simulink model "PID_validation_3_3_2"  (R2024b)
settings: Solver=FixedStepDiscrete  StartTime=0.0  StopTime=20  FixedStep=0.001  RelTol=1e-3
undefined symbols (not defined in the file): degs2rpm, DiscIntNeverNeededParam, K_W, kd, ki, kp, National_Instruments, PCI, rdp, sens, step_gain, tl, Ts, u_bar_max
libraries: sldrtlib x3, simulink x1
settings Model: SimulationMode=external  ExtModeTrigDuration=20001  Creator=fasoloandr  LastModifiedBy=Enrico 2
settings DataIOCC: ReturnWorkspaceOutputs=off
settings HardwareCC: ProdBitPerLong=64  ProdHWDeviceType=Intel->x86-64 (Linux 64)
settings RTWCC: Description=Simulink Desktop Real-Time  SystemTargetFile=sldrt.tlc  TemplateMakefile=sldrt.tmf  RTWCompilerOptimization=on
settings CodeAppCC: MaxIdLength=95
settings SimulinkDesktopRealTimeCC: TargetLibSuffix=_sldrt.a  TargetPreCompLibLocation=C:\Program Files\MATLAB\R2024b\toolbox\sldrt\lib\win64  ParMdlRefBuildCompliant=on

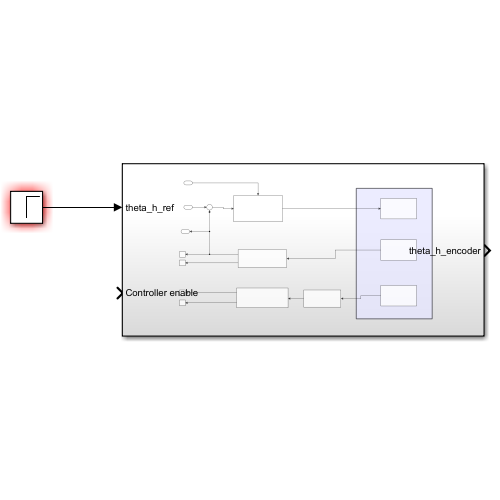
[thumbnail: Simulink's stored preview of the top-level diagram]
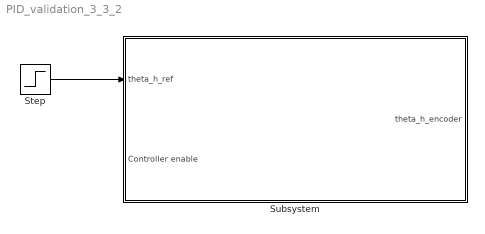
== system PID_validation_3_3_2 ==
  Step : Step  After=step_gain  SampleTime=0
  Subsystem : Subsystem
  wires:
  Step/1 -> Subsystem/1(theta_h_ref)

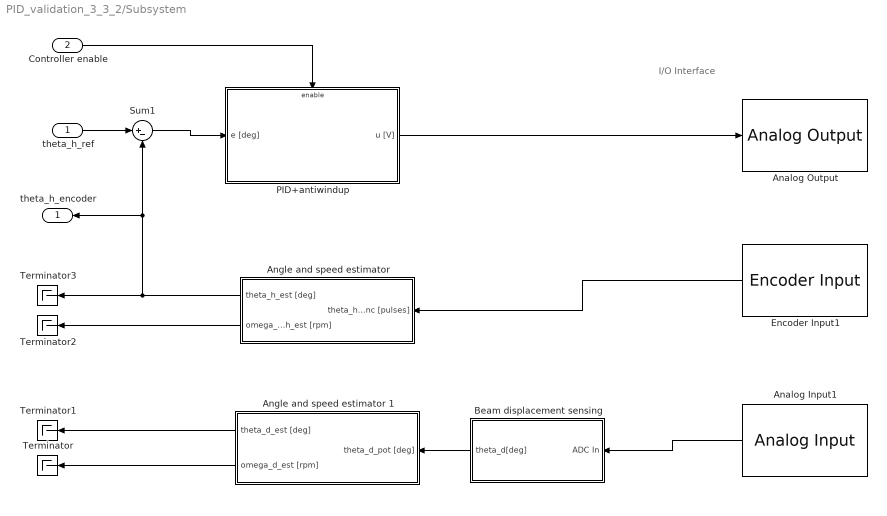
== system PID_validation_3_3_2/Subsystem ==
  note: I/O Interface
  theta_h_ref : Inport
  Controller enable : Inport  Port=2
  Analog Input1 : sldrtlib/Analog Input  SampleTime=-1  MaxMissedTicks=10  ShowMissedTicks=off  YieldWhenWaiting=off  DrvName=National_Instruments/PCI-6221  DrvAddress=4294967295  DrvOptions=[0 0 0 2 0]  Channels=[1,2]  RangeMode=1  VoltRange=1  DataType=1
      settings: AttributesFormatString=National Instruments\nPCI-6221 [auto]
  Analog Output : sldrtlib/Analog Output  SampleTime=-1  MaxMissedTicks=10  ShowMissedTicks=off  YieldWhenWaiting=off  DrvName=National_Instruments/PCI-6221  DrvAddress=4294967295  DrvOptions=[0 0 0 2 0]  Channels=1  RangeMode=1  VoltRange=1  InitialValue=[0]  FinalValue=[0]
      settings: AttributesFormatString=National Instruments\nPCI-6221 [auto]
  Angle and speed estimator : Subsystem
  Angle and speed estimator 1 : Subsystem
  Beam displacement sensing : Subsystem
  Encoder Input1 : sldrtlib/Encoder Input  SampleTime=-1  MaxMissedTicks=10  ShowMissedTicks=off  YieldWhenWaiting=off  DrvName=National_Instruments/PCI-6221  DrvAddress=4294967295  DrvOptions=[0 0 0 2 0]  Channels=1  QuadMode=3  IndexPulse=1  InputFilter=Inf  DataType=1
      settings: AttributesFormatString=National Instruments\nPCI-6221 [auto]
  PID+antiwindup : Subsystem
  Sum1 : Sum  Inputs=|+-
  Terminator{,1..3} (4 alike) : Terminator
  theta_h_encoder : Outport
  wires:
  Angle and speed estimator/1(theta_h_est [deg]) -> theta_h_encoder/1, Sum1/2, Terminator3/1
  Angle and speed estimator/2(omega_h_est [rpm]) -> Terminator2/1
  Angle and speed estimator 1/2(omega_d_est [rpm]) -> Terminator/1
  theta_h_ref/1 -> Sum1/1
  Sum1/1 -> PID+antiwindup/1(e [deg])
  Encoder Input1/1 -> Angle and speed estimator/1(theta_h_enc [pulses])
  Analog Input1/1 -> Beam displacement sensing/1(ADC In)
  PID+antiwindup/1(u [V]) -> Analog Output/1
  Angle and speed estimator 1/1(theta_d_est [deg]) -> Terminator1/1
  Beam displacement sensing/1(theta_d[deg]) -> Angle and speed estimator 1/1(theta_d_pot [deg])
  Controller enable/1 -> PID+antiwindup/Enable

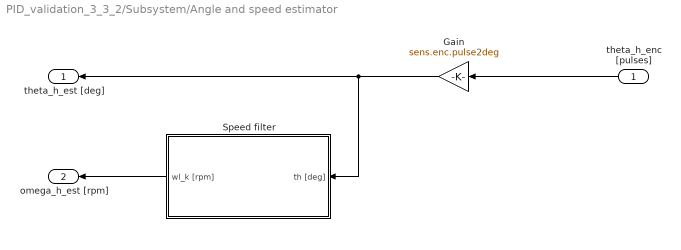
== system PID_validation_3_3_2/Subsystem/Angle and speed estimator ==
  theta_h_enc [pulses] : Inport
  Gain : Gain  Gain=sens.enc.pulse2deg
  Speed filter : Subsystem
  theta_h_est [deg] : Outport
  omega_h_est [rpm] : Outport  Port=2
  wires:
  Speed filter/1(wl_k [rpm]) -> omega_h_est [rpm]/1
  theta_h_enc [pulses]/1 -> Gain/1
  Gain/1 -> Speed filter/1(th [deg]), theta_h_est [deg]/1

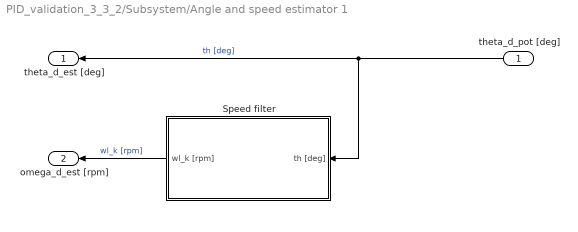
== system PID_validation_3_3_2/Subsystem/Angle and speed estimator 1 ==
  theta_d_pot [deg] : Inport
  Speed filter : Subsystem
  theta_d_est [deg] : Outport
  omega_d_est [rpm] : Outport  Port=2
  wires:
  Speed filter/1(wl_k [rpm]) -> omega_d_est [rpm]/1  "wl_k [rpm]"
  theta_d_pot [deg]/1 -> Speed filter/1(th [deg]), theta_d_est [deg]/1  "th [deg]"

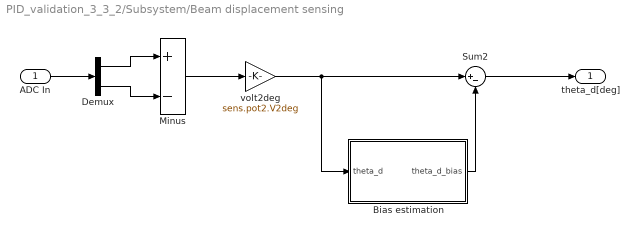
== system PID_validation_3_3_2/Subsystem/Beam displacement sensing ==
  ADC In : Inport
  " Bias estimation" : Subsystem
  Demux : Demux  Outputs=2
  Minus : Sum  Inputs=+-
  Sum2 : Sum  Inputs=|+-
  volt2deg : Gain  Gain=sens.pot2.V2deg
  theta_d[deg] : Outport
  wires:
  volt2deg/1 -> " Bias estimation"/1(theta_d), Sum2/1
  Sum2/1 -> theta_d[deg]/1
  " Bias estimation"/1(theta_d_bias) -> Sum2/2
  Minus/1 -> volt2deg/1
  Demux/2 -> Minus/2
  ADC In/1 -> Demux/1
  Demux/1 -> Minus/1

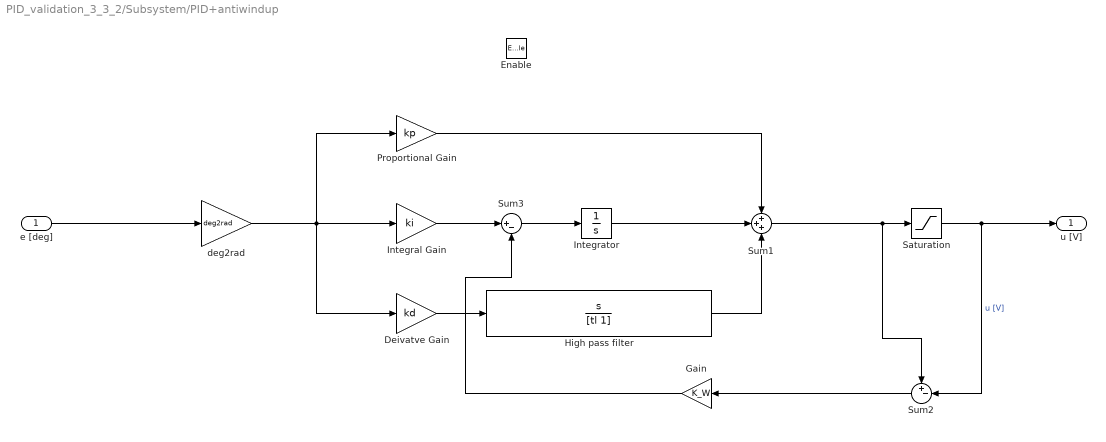
== system PID_validation_3_3_2/Subsystem/PID+antiwindup ==
  e [deg] : Inport
  Enable : EnablePort
  Deivatve Gain : Gain  Gain=kd
  Gain : Gain  Gain=K_W
  High pass filter : TransferFcn  Numerator=[1 0]  Denominator=[tl 1]
  Integral Gain : Gain  Gain=ki
  Integrator : Integrator
  Proportional Gain : Gain  Gain=kp
  "Saturation " : Saturate  UpperLimit=u_bar_max  LowerLimit=-u_bar_max
  Sum1 : Sum  Inputs=+++
  Sum2 : Sum  Inputs=+-|
  Sum3 : Sum  Inputs=|+-
  deg2rad : Gain  Gain=deg2rad
  u [V] : Outport
  wires:
  Integrator/1 -> Sum1/2
  e [deg]/1 -> deg2rad/1
  Sum3/1 -> Integrator/1
  Sum1/1 -> Sum2/1, "Saturation "/1
  Sum2/1 -> Gain/1
  Proportional Gain/1 -> Sum1/1
  deg2rad/1 -> Deivatve Gain/1, Proportional Gain/1, Integral Gain/1
  High pass filter/1 -> Sum1/3
  Integral Gain/1 -> Sum3/1
  "Saturation "/1 -> Sum2/2, u [V]/1  "u [V]"
  Deivatve Gain/1 -> High pass filter/1
  Gain/1 -> Sum3/2

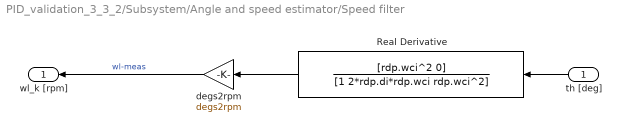
== system PID_validation_3_3_2/Subsystem/Angle and speed estimator/Speed filter ==
  th [deg] : Inport
  Real Derivative : TransferFcn  Numerator=[rdp.wci^2 0]  Denominator=[1 2*rdp.di*rdp.wci rdp.wci^2]
  degs2rpm : Gain  Gain=degs2rpm
  wl_k [rpm] : Outport
  wires:
  th [deg]/1 -> Real Derivative/1
  degs2rpm/1 -> wl_k [rpm]/1  "wl-meas"
  Real Derivative/1 -> degs2rpm/1

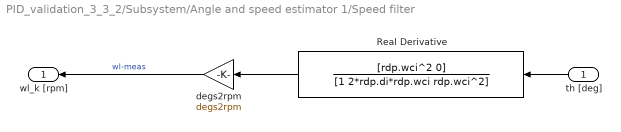
== system PID_validation_3_3_2/Subsystem/Angle and speed estimator 1/Speed filter ==
  th [deg] : Inport
  Real Derivative : TransferFcn  Numerator=[rdp.wci^2 0]  Denominator=[1 2*rdp.di*rdp.wci rdp.wci^2]
  degs2rpm : Gain  Gain=degs2rpm
  wl_k [rpm] : Outport
  wires:
  th [deg]/1 -> Real Derivative/1
  degs2rpm/1 -> wl_k [rpm]/1  "wl-meas"
  Real Derivative/1 -> degs2rpm/1

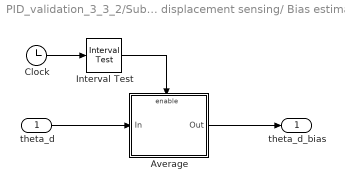
== system PID_validation_3_3_2/Subsystem/Beam displacement sensing/ Bias estimation ==
  theta_d : Inport
  Average : Subsystem
  Clock : Clock
  Interval Test : simulink/Logic and Bit Operations/Interval Test  IntervalClosedRight=on  uplimit=0.5  IntervalClosedLeft=on  lowlimit=-0.5  OutDataTypeStr=boolean
  theta_d_bias : Outport
  wires:
  Clock/1 -> Interval Test/1
  theta_d/1 -> Average/1(In)
  Interval Test/1 -> Average/Enable
  Average/1(Out) -> theta_d_bias/1

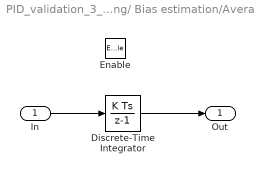
== system PID_validation_3_3_2/Subsystem/Beam displacement sensing/ Bias estimation/Average ==
  In : Inport
  Enable : EnablePort
  Discrete-Time Integrator : DiscreteIntegrator  SampleTime=Ts  ICPrevOutput=DiscIntNeverNeededParam  ICPrevScaledInput=DiscIntNeverNeededParam
  Out : Outport
  wires:
  In/1 -> Discrete-Time Integrator/1
  Discrete-Time Integrator/1 -> Out/1
